simulink model "myGuyton_corrected_new"  (Simulink 6.6)
settings: Solver=ode15s  StartTime=0  StopTime=60*24*14  FixedStep=0.025  MaxStep=1  MinStep=0.00000001  RelTol=1e-1
values from neighbouring files (symbols this model uses):
  A1K = 0.5    [G92_var_decl_exp.m]
  A2K = 60    [G92_var_decl_exp.m]
  A3K = 40000    [G92_var_decl_exp.m]
  A4K = 0.1    [G92_var_decl_exp.m]
  A4K2 = 40000    [G92_var_decl_exp.m]
  AARK = 1    [G92_var_decl_exp.m]
  AARLL = 4    [G92_var_decl_exp.m]
  ADHC_IC = 1.01449    [G92_var_decl_exp.m]
  ADHINF = 0    [G92_var_decl_exp.m]
  ADHKLL = 0.2    [G92_var_decl_exp.m]
  ADHKUL = 5    [G92_var_decl_exp.m]
  ADHPAM = 0.3    [G92_var_decl_exp.m]
  ADHPUL = 85    [G92_var_decl_exp.m]
  ADHTC = 15    [G92_var_decl_exp.m]
  ADHVLL = 0.93617    [G92_var_decl_exp.m]
  ADHVUL = 2.5    [G92_var_decl_exp.m]
  AH10 = 0.333    [G92_var_decl_exp.m]
  AH11 = 1000    [G92_var_decl_exp.m]
  AH9 = 1    [G92_var_decl_exp.m]
  AHMNAR = 0.3    [G92_var_decl_exp.m]
  AHTHM = 2    [G92_var_decl_exp.m]
  AHY_IC = -0.461862    [G92_var_decl_exp.m]
  ALCLK = 0.3    [G92_var_decl_exp.m]
  ALDINF = 0    [G92_var_decl_exp.m]
  ALDKNS = 0    [G92_var_decl_exp.m]
  ALDMM = 2.5    [G92_var_decl_exp.m]
  AM1LL = 0    [G92_var_decl_exp.m]
  AM1UL = 5    [G92_var_decl_exp.m]
  AMC_IC = 1.05537    [G92_var_decl_exp.m]
  AMCSNS = 0.65    [G92_var_decl_exp.m]
  AMKM = 0.5    [G92_var_decl_exp.m]
  AMKMUL = 12    [G92_var_decl_exp.m]
  AMM1_IC = 1.00227    [G92_var_decl_exp.m]
  AMM2_IC = 1.09458    [G92_var_decl_exp.m]
  AMM4 = 0.005    [G92_var_decl_exp.m]
  AMNALL = 0.04    [G92_var_decl_exp.m]
  AMNAM = 0.8    [G92_var_decl_exp.m]
  AMNAUL = 15    [G92_var_decl_exp.m]
  AMT = 60    [G92_var_decl_exp.m]
  ANC_IC = 0.867681    [G92_var_decl_exp.m]
  ANCSNS = 0.4    [G92_var_decl_exp.m]
  ANGINF = 0    [G92_var_decl_exp.m]
  ANGKNS = 0    [G92_var_decl_exp.m]
  ANMALD = 2.5    [G92_var_decl_exp.m]
  ANMAM = 1.4    [G92_var_decl_exp.m]
  ANMARL = 0.86    [G92_var_decl_exp.m]
  ANMEM = 1.6    [G92_var_decl_exp.m]
  ANMKEL = 0.3    [G92_var_decl_exp.m]
  ANMKEM = 2    [G92_var_decl_exp.m]
  ANMLL = 0.7    [G92_var_decl_exp.m]
  ANMNAM = 1    [G92_var_decl_exp.m]
  ANMSLT = 2    [G92_var_decl_exp.m]
  ANMTM = 1.5    [G92_var_decl_exp.m]
  ANMUL = 1.8    [G92_var_decl_exp.m]
  ANPC_IC = 0.9333    [G92_var_decl_exp.m]
  ANPINF = 0    [G92_var_decl_exp.m]
  ANPKNS = 0    [G92_var_decl_exp.m]
  ANPTC = 4    [G92_var_decl_exp.m]
  ANPXAF = 1.5    [G92_var_decl_exp.m]
  ANPXUL = 10    [G92_var_decl_exp.m]
  ANT = 12    [G92_var_decl_exp.m]
  ANULL = 0.8    [G92_var_decl_exp.m]
  ANUM = 6    [G92_var_decl_exp.m]
  ANUVM = 0    [G92_var_decl_exp.m]
  ANV = 5000    [G92_var_decl_exp.m]
  ANX1_IC = 0    [G92_var_decl_exp.m]
  ANXM = 0    [G92_var_decl_exp.m]
  ANY = -0.2    [G92_var_decl_exp.m]
  AR1_IC = 1.00197    [G92_var_decl_exp.m]
  AR2_IC = 1.00306    [G92_var_decl_exp.m]
  AR3_IC = 1.05777    [G92_var_decl_exp.m]
  ARF = 0.5    [G92_var_decl_exp.m]
  ATRFBM = 0    [G92_var_decl_exp.m]
  ATRVM = 0    [G92_var_decl_exp.m]
  AU1_IC = 0.99999    [G92_var_decl_exp.m]
  AU4_IC = -0.00833091    [G92_var_decl_exp.m]
  AU6_IC = 1.00041    [G92_var_decl_exp.m]
  AUC1 = 0.3    [G92_var_decl_exp.m]
  AUDMP = 0.3    [G92_var_decl_exp.m]
  AUK = 0.004    [G92_var_decl_exp.m]
  AUL = 1.5    [G92_var_decl_exp.m]
  AULPM = 0    [G92_var_decl_exp.m]
  AUM1 = 3    [G92_var_decl_exp.m]
  AUM2 = 1    [G92_var_decl_exp.m]
  AUMAX = 5    [G92_var_decl_exp.m]
  AUMIN = 0.4    [G92_var_decl_exp.m]
  AUMK1 = 0.3    [G92_var_decl_exp.m]
  AUN1 = 0.5    [G92_var_decl_exp.m]
  AUS = 1    [G92_var_decl_exp.m]
  AUSLP = 1.5    [G92_var_decl_exp.m]
  AUTOGN = 7    [G92_var_decl_exp.m]
  AUTOK = 0.1    [G92_var_decl_exp.m]
  AUTOSN = 0.9    [G92_var_decl_exp.m]
  AUV = 0.55    [G92_var_decl_exp.m]
  AUX = 1    [G92_var_decl_exp.m]
  AUY = 0    [G92_var_decl_exp.m]
  BAROTC = 0.16    [G92_var_decl_exp.m]
  CFC = 0.01167    [G92_var_decl_exp.m]
  CKEEX = 4    [G92_var_decl_exp.m]
  CMPTSS = 2    [G92_var_decl_exp.m]
  CN2 = 0.0212    [G92_var_decl_exp.m]
  CN3_IC = 0.359907    [G92_var_decl_exp.m]
  CN7 = 0.2    [G92_var_decl_exp.m]
  CNR = 139    [G92_var_decl_exp.m]
  CPF = 0.0003    [G92_var_decl_exp.m]
  CPK = 0.000253    [G92_var_decl_exp.m]
  CPR = 40    [G92_var_decl_exp.m]
  CRRFLX = 0    [G92_var_decl_exp.m]
  CV = 0.1    [G92_var_decl_exp.m]
  DFP_IC = 1.16492e-06    [G92_var_decl_exp.m]
  DHDTR = 0.05    [G92_var_decl_exp.m]
  DIURET = 1    [G92_var_decl_exp.m]
  DR = 0    [G92_var_decl_exp.m]
  DTKA_IC = 0.0368507    [G92_var_decl_exp.m]
  DTNAR = 0.675    [G92_var_decl_exp.m]
  DTNARL = 1e-06    [G92_var_decl_exp.m]
  EARK = 1    [G92_var_decl_exp.m]
  EARLL = 24    [G92_var_decl_exp.m]
  EFAFR = 0    [G92_var_decl_exp.m]
  EXC = 1    [G92_var_decl_exp.m]
  ... (+137 more)
libraries: simulink x5
(part 2 of 3)

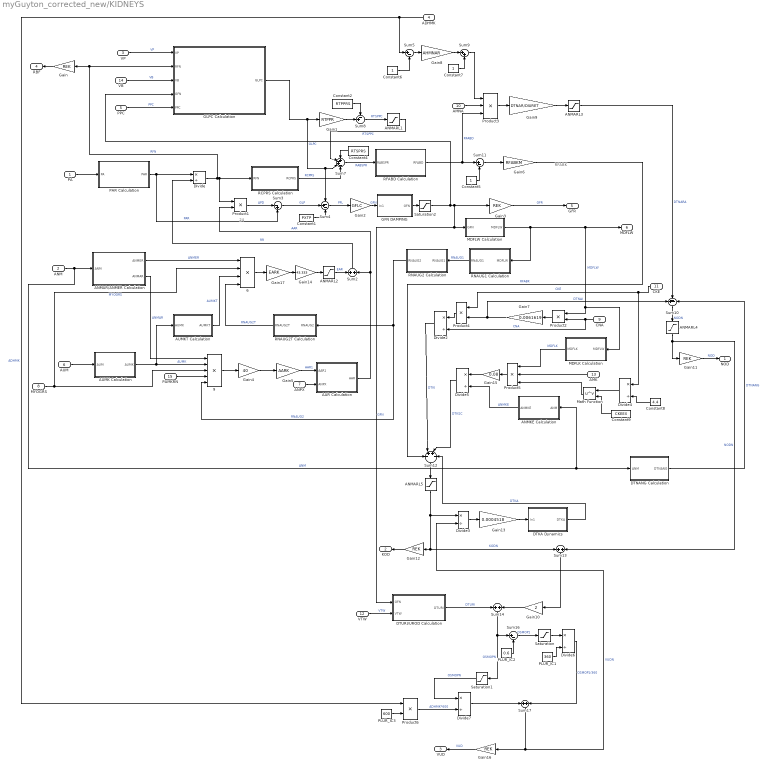
== system myGuyton_corrected_new/KIDNEYS ==
  note: RFABK
  note: 24
  PA : Inport
  ANM : Inport  Port=2
  VP : Inport  Port=3
  ADHMK : Inport  Orientation=left  Port=4
  PPC : Inport  Port=5
  AUM : Inport  Port=6
  ANPX : Inport  Port=7
  MYOGRS : Inport  Port=8
  CNA : Inport  Orientation=left  Port=9
  AMNA : Inport  Port=10
  CKE : Inport  Orientation=left  Port=11
  VTW : Inport  Port=12
  AMK : Inport  Orientation=left  Port=13
  VB : Inport  Port=14
  PAMKRN : Inport  Port=15
  6 : Product  Inputs=4  RndMeth=Zero
  9 : Product  Inputs=5  RndMeth=Zero
  AAR Calculation : Subsystem
  ANMAR/ANMER Calculation : Subsystem
  ANMARL1 : Saturate  UpperLimit=inf  LowerLimit=1
  ANMARL2 : Saturate  UpperLimit=inf  LowerLimit=EARLL
  ANMARL3 : Saturate  UpperLimit=inf  LowerLimit=DTNARL
  ANMARL4 : Saturate  Orientation=down  UpperLimit=inf  LowerLimit=0.00000001
  ANMARL5 : Saturate  Orientation=down  UpperLimit=inf  LowerLimit=0
  ANMKE Calculation : Subsystem  Orientation=left
  AUMK Calculation : Subsystem
  AUMKT Calculation : Subsystem
  Constant1 : Constant  Value=PXTP
  Constant2 : Constant  Value=RTPPRS
  Constant4 : Constant  Orientation=left  Value=RTSPRS
  Constant5 : Constant
  Constant6 : Constant
  Constant7 : Constant
  Constant8 : Constant  Orientation=left  Value=4.4
  Constant9 : Constant  Orientation=left  Value=CKEEX
  DTKA Dynamics : Subsystem
      mask Display: dpoly([0 1],[1 1])
  DTNANG Calculation : Subsystem
  DTURI/UROD Calculation : Subsystem
  Divide{,3,6..7} (4 alike) : Product  Inputs=*/  OutScaling=2^-10
  Divide2 : Product  Orientation=left  Inputs=*/  OutScaling=2^-10
  Divide4 : Product  Orientation=left  Inputs=*/  OutScaling=2^-10
  Divide5 : Product  Orientation=left  Inputs=*/  OutScaling=2^-10
  GFN DAMPING : Subsystem
      mask Display: dpoly([0 1],[GFNDMP 1])
  GLPC Calculation : Subsystem
  Gain : Gain  Orientation=left  Gain=REK
  Gain1 : Gain  Gain=RTPPR
  Gain10 : Gain  Orientation=left  Gain=2
  Gain11 : Gain  Gain=REK
  Gain12 : Gain  Orientation=left  Gain=REK
  Gain13 : Gain  Gain=0.0004518
  Gain14 : Gain  Gain=43.333
  Gain15 : Gain  Orientation=left  Gain=0.08
  Gain16 : Gain  Orientation=left  Gain=REK
  Gain17 : Gain  Gain=EARK
  Gain2 : Gain  Gain=GFLC
  Gain3 : Gain  Gain=REK
  Gain4 : Gain  Gain=40
  Gain5 : Gain  Gain=AARK
  Gain6 : Gain  Gain=RFABKM
  Gain7 : Gain  Orientation=left  Gain=0.0061619
  Gain8 : Gain  Gain=AHMNAR
  Gain9 : Gain  Gain=DTNAR/DIURET
  MDFLK Calculation : Subsystem  Orientation=left
  MDFLW Calculation : Subsystem
  Math Function : Math  Orientation=left  Operator=pow  SaturateOnIntegerOverflow=on
  PAR Calculation : Subsystem
  PLUR_IC1 : Constant  Value=360
  PLUR_IC2 : Constant  Value=0.6
  PLUR_IC3 : Constant  Value=600
  Product1 : Product  RndMeth=Zero
  Product2 : Product  Orientation=left  RndMeth=Zero
  Product3 : Product  Inputs=3  RndMeth=Zero
  Product4 : Product  Orientation=left  RndMeth=Zero
  Product5 : Product  Orientation=left  Inputs=3  RndMeth=Zero
  Product6 : Product  RndMeth=Zero
  RCPRS Calculation : Subsystem
  RFABD Calculation : Subsystem
  RNAUG1 Calculation : Subsystem  Orientation=left
  RNAUG2 Calculation : Subsystem  Orientation=left
  RNAUG2T Calculation : Subsystem  Orientation=left
  Saturation : Saturate  UpperLimit=inf  LowerLimit=0
  Saturation1 : Saturate  Orientation=left  UpperLimit=0.6  LowerLimit=-inf
  Saturation2 : Saturate  UpperLimit=inf  LowerLimit=GFNLL
  Sum10 : Sum  Orientation=down  Inputs=+--
  Sum11 : Sum  Inputs=|+-
  Sum12 : Sum  Orientation=down  Inputs=-++-
  Sum13 : Sum  Orientation=down
  Sum14 : Sum  Orientation=down
  Sum16 : Sum  Inputs=|+-
  Sum17 : Sum  Orientation=down
  Sum2 : Sum  Orientation=up
  Sum3 : Sum  Inputs=|-+
  Sum4 : Sum  Inputs=-+-
  Sum5 : Sum  Inputs=|+-
  Sum7 : Sum  Inputs=+-+-
  Sum8 : Sum  Inputs=-+|
  Sum9 : Sum  Inputs=|++
  NOD : Outport
  KOD : Outport  Orientation=left  Port=2
  VUD : Outport  Orientation=left  Port=3
  RBF : Outport  Orientation=left  Port=4
  GFR : Outport  Port=5
  MDFLW : Outport  Port=6
  wires:
  PAR Calculation/1(PAR) -> Divide/1, Sum3/2  "PAR"
  PA/1 -> PAR Calculation/1(PA)
  Divide/1 -> RCPRS Calculation/1(RFN), Product1/1, Gain/1, GLPC Calculation/2(RFN)  "RFN"
  Gain/1 -> RBF/1
  ANMAR/ANMER Calculation/1(ANMER) -> 6/1  "ANMER"
  RCPRS Calculation/1(RCPRS) -> Sum7/4  "RCPRS"
  AUM/1 -> AUMK Calculation/1(AUM)
  AUMK Calculation/1(AUMK) -> 9/2, AUMKT Calculation/1(AUMK)  "AUMK"
  GLPC Calculation/1(GLPC) -> Gain1/1, Sum7/3, Sum4/1  "GLPC"
  Constant2/1 -> Sum8/1
  Gain1/1 -> Sum8/2
  Sum8/1 -> ANMARL1/1  "RTSPPC"
  ANMARL1/1 -> Sum7/2  "RTSPPC"
  Constant4/1 -> Sum7/1
  Sum7/1 -> RFABD Calculation/1(RABSPR)  "RABSPR"
  RFABD Calculation/1(RFABD) -> Sum11/1, Product3/3  "RFABD"
  Sum11/1 -> Gain6/1
  Constant5/1 -> Sum11/2
  Gain6/1 -> Sum12/1  "RFABK"
  ANMAR/ANMER Calculation/2(ANMAR) -> 9/1  "ANMAR"
  9/1 -> Gain4/1
  Gain4/1 -> Gain5/1
  Gain5/1 -> AAR Calculation/1(AAR1)  "AAR1"
  MYOGRS/1 -> 9/3, 6/2  "MYOGRS"
  AAR Calculation/1(AAR) -> Product1/2, Sum2/2  "AAR"
  ANPX/1 -> AAR Calculation/2(ANPX)
  ANM/1 -> ANMAR/ANMER Calculation/1(ANM), ANMKE Calculation/1(ANM), DTNANG Calculation/1(ANM)  "ANM"
  AUMKT Calculation/1(AUMKT) -> 6/3  "AUMKT"
  RNAUG2T Calculation/1(RNAUG2T) -> 6/4  "RNAUG2T"
  ANMARL2/1 -> Sum2/1  "EAR"
  Sum2/1 -> Divide/2  "RR"
  Product1/1 -> Sum3/1  "APD"
  Sum3/1 -> Sum4/2  "GLP"
  Constant1/1 -> Sum4/3
  Sum4/1 -> Gain2/1  "PFL"
  Gain2/1 -> GFN DAMPING/1(In1)  "GFN"
  Gain3/1 -> GFR/1  "GFR"
  MDFLW Calculation/1(MDFLW) -> RNAUG1 Calculation/1(MDFLW), MDFLW/1, Product2/1, MDFLK Calculation/1(MDFLW)  "MDFLW"
  RNAUG1 Calculation/1(RNAUG1) -> RNAUG2 Calculation/1(RNAUG1)  "RNAUG1"
  RNAUG2 Calculation/1(RNAUG2) -> RNAUG2T Calculation/1(RNAUG2), 9/5  "RNAUG2"
  CNA/1 -> Product2/2, Divide2/2  "CNA"
  Product2/1 -> Gain7/1
  Gain7/1 -> Product4/2, Sum10/1  "DTNAI"
  AMNA/1 -> Product3/2
  ADHMK/1 -> Sum5/1, Product6/1  "ADHMK"
  Constant6/1 -> Sum5/2
  Sum5/1 -> Gain8/1
  Gain8/1 -> Sum9/1
  Constant7/1 -> Sum9/2
  Sum9/1 -> Product3/1
  Product3/1 -> Gain9/1
  Gain9/1 -> ANMARL3/1
  CKE/1 -> Product4/1, Divide4/1  "CKE"
  Product4/1 -> Divide2/1
  Divide2/1 -> Sum12/2  "DTKI"
  ANMARL3/1 -> Sum10/2  "DTNARA"
  Sum10/1 -> ANMARL4/1  "NODN"
  Gain11/1 -> NOD/1  "NOD"
  Divide5/1 -> Sum12/3  "DTKSC"
  Sum12/1 -> ANMARL5/1
  ANMARL5/1 -> Sum13/1, Gain12/1, Divide3/1  "KODN"
  DTNANG Calculation/1(DTNANG) -> Sum10/3  "DTNANG"
  Sum13/1 -> Gain10/1
  Gain12/1 -> KOD/1
  Gain10/1 -> Sum14/2
  Divide3/1 -> Gain13/1
  Gain13/1 -> DTKA Dynamics/1(In1)
  DTKA Dynamics/1(DTKA) -> Sum12/4  "DTKA"
  Sum14/1 -> Sum16/1, Saturation1/1  "OSMOPN"
  PLUR_IC2/1 -> Sum16/2
  Sum16/1 -> Saturation/1  "OSMOP1"
  Saturation1/1 -> Divide7/1  "OSMOPN"
  Saturation/1 -> Divide6/1
  PLUR_IC1/1 -> Divide6/2
  Divide6/1 -> Sum17/2  "OSMOP1/360"
  Sum17/1 -> Divide3/2, Gain16/1  "VUDN"
  PLUR_IC3/1 -> Product6/2
  Product6/1 -> Divide7/2  "ADHMK*600"
  Divide7/1 -> Sum17/1
  Gain16/1 -> VUD/1  "VUD"
  DTURI/UROD Calculation/1(DTURI) -> Sum14/1  "DTURI"
  VTW/1 -> DTURI/UROD Calculation/2(VTW)  "VTW"
  Constant8/1 -> Divide4/2
  Divide4/1 -> Math Function/1
  Constant9/1 -> Math Function/2
  Math Function/1 -> Product5/3
  AMK/1 -> Product5/2
  MDFLK Calculation/1(MDFLK) -> Product5/1  "MDFLK"
  Product5/1 -> Gain15/1
  Gain15/1 -> Divide5/1
  ANMKE Calculation/1(ANMKE) -> Divide5/2  "ANMKE"
  VP/1 -> GLPC Calculation/1(VP)  "VP"
  VB/1 -> GLPC Calculation/3(VB)  "VB"
  PPC/1 -> GLPC Calculation/5(PPC)  "PPC"
  PAMKRN/1 -> 9/4
  Gain14/1 -> ANMARL2/1
  6/1 -> Gain17/1
  Gain17/1 -> Gain14/1
  ANMARL4/1 -> Sum13/2, Gain11/1  "NODN"
  Saturation2/1 -> Gain3/1, MDFLW Calculation/1(GFN), DTURI/UROD Calculation/1(GFN), GLPC Calculation/4(GFN)  "GFN"
  GFN DAMPING/1(GFN) -> Saturation2/1

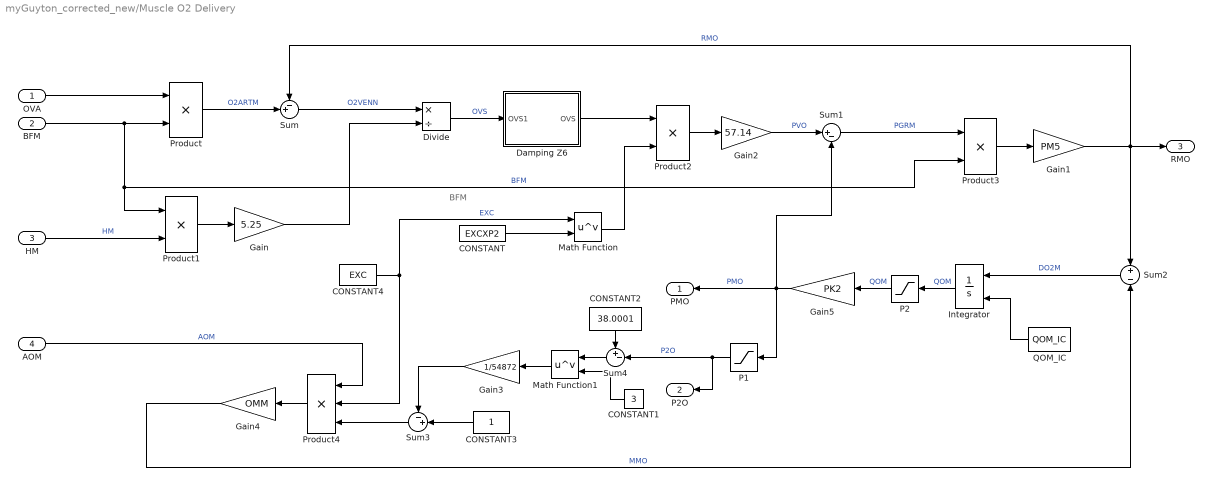
== system myGuyton_corrected_new/Muscle O2 Delivery ==
  note: BFM
  OVA : Inport
  BFM : Inport  Port=2
  HM : Inport  Port=3
  AOM : Inport  Port=4
  CONSTANT : Constant  Value=EXCXP2
  CONSTANT1 : Constant  Orientation=left  Value=3
  CONSTANT2 : Constant  Orientation=down  Value=38.0001
  CONSTANT3 : Constant  Orientation=left
  CONSTANT4 : Constant  Value=EXC
  Damping Z6 : Subsystem
      mask Display: dpoly([0 1], [Z6 1])
  Divide : Product  Inputs=*/  OutScaling=2^-10
  Gain : Gain  Gain=5.25
  Gain1 : Gain  Gain=PM5
  Gain2 : Gain  Gain=57.14
  Gain3 : Gain  Orientation=left  Gain=1/54872
  Gain4 : Gain  Orientation=left  Gain=OMM
  Gain5 : Gain  Orientation=left  Gain=PK2
  Integrator : Integrator  Orientation=left  InitialConditionSource=external
  Math Function : Math  Operator=pow  SaturateOnIntegerOverflow=on
  Math Function1 : Math  Orientation=left  Operator=pow  SaturateOnIntegerOverflow=on
  P1 : Saturate  Orientation=left  UpperLimit=38  LowerLimit=-inf
  P2 : Saturate  Orientation=left  UpperLimit=inf  LowerLimit=0.0001
  Product{,1..3} (4 alike) : Product  RndMeth=Zero
  Product4 : Product  Orientation=left  Inputs=3  RndMeth=Zero
  QOM_IC : Constant  Orientation=left  Value=QOM_IC
  Sum : Sum  Inputs=-+|
  Sum1 : Sum  Inputs=|+-
  Sum2 : Sum  Orientation=left  Inputs=+-
  Sum3 : Sum  Orientation=left  Inputs=-+|
  Sum4 : Sum  Orientation=left  Inputs=+-|
  PMO : Outport  Orientation=left
  P2O : Outport  Orientation=left  Port=2
  RMO : Outport  Port=3
  wires:
  Divide/1 -> Damping Z6/1(OVS1)  "OVS"
  Product/1 -> Sum/2  "O2ARTM"
  Sum/1 -> Divide/1  "O2VENN"
  Gain/1 -> Divide/2
  Product1/1 -> Gain/1
  HM/1 -> Product1/2  "HM"
  BFM/1 -> Product/2, Product1/1, Product3/2  "BFM"
  OVA/1 -> Product/1
  CONSTANT/1 -> Math Function/2
  Math Function/1 -> Product2/2
  Product2/1 -> Gain2/1
  Product3/1 -> Gain1/1
  Gain1/1 -> Sum/1, Sum2/1, RMO/1  "RMO"
  Sum2/1 -> Integrator/1  "DO2M"
  QOM_IC/1 -> Integrator/2
  Integrator/1 -> P2/1  "QOM"
  P2/1 -> Gain5/1  "QOM"
  Gain5/1 -> Sum1/2, PMO/1, P1/1  "PMO"
  Gain2/1 -> Sum1/1  "PVO"
  Sum1/1 -> Product3/1  "PGRM"
  P1/1 -> Sum4/2, P2O/1  "P2O"
  CONSTANT2/1 -> Sum4/1
  Sum4/1 -> Math Function1/1
  CONSTANT1/1 -> Math Function1/2
  Math Function1/1 -> Gain3/1
  CONSTANT3/1 -> Sum3/2
  Gain3/1 -> Sum3/1
  Sum3/1 -> Product4/3
  AOM/1 -> Product4/1  "AOM"
  Product4/1 -> Gain4/1
  Gain4/1 -> Sum2/2  "MMO"
  CONSTANT4/1 -> Math Function/1, Product4/2  "EXC"
  Damping Z6/1(OVS) -> Product2/1

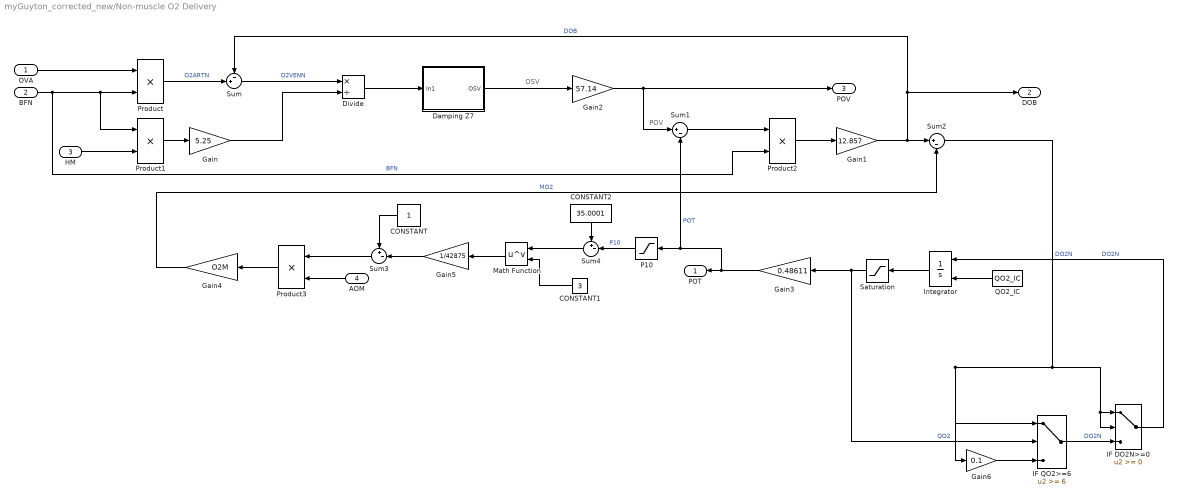
== system myGuyton_corrected_new/Non-muscle O2 Delivery ==
  note: POV
  note: OSV
  OVA : Inport
  BFN : Inport  Port=2
  HM : Inport  Port=3
  AOM : Inport  Orientation=left  Port=4
  CONSTANT : Constant  Orientation=left
  CONSTANT1 : Constant  Orientation=left  Value=3
  CONSTANT2 : Constant  Orientation=down  Value=35.0001
  Damping Z7 : Subsystem
      mask Display: dpoly([0 1], [Z7 1])
  Divide : Product  Inputs=*/  OutScaling=2^-10
  Gain : Gain  Gain=5.25
  Gain1 : Gain  Gain=12.857
  Gain2 : Gain  Gain=57.14
  Gain3 : Gain  Orientation=left  Gain=0.48611
  Gain4 : Gain  Orientation=left  Gain=O2M
  Gain5 : Gain  Orientation=left  Gain=1/42875
  Gain6 : Gain  Gain=0.1
  IF DO2N>=0 : Switch
  IF QO2>=6 : Switch  Threshold=6
  Integrator : Integrator  Orientation=left  InitialConditionSource=external
  Math Function : Math  Orientation=left  Operator=pow  SaturateOnIntegerOverflow=on
  P10 : Saturate  Orientation=left  UpperLimit=35  LowerLimit=-inf
  Product : Product  RndMeth=Zero
  Product1 : Product  RndMeth=Zero
  Product2 : Product  RndMeth=Zero
  Product3 : Product  Orientation=left  RndMeth=Zero
  QO2_IC : Constant  Orientation=left  Value=QO2_IC
  Saturation : Saturate  Orientation=left  UpperLimit=inf  LowerLimit=0
  Sum : Sum  Inputs=-+|
  Sum1 : Sum  Inputs=|+-
  Sum2 : Sum  Inputs=|+-
  Sum3 : Sum  Orientation=left  Inputs=+-|
  Sum4 : Sum  Orientation=left  Inputs=+-|
  POT : Outport  Orientation=left
  DOB : Outport  Port=2
  POV : Outport  Port=3
  wires:
  OVA/1 -> Product/1
  BFN/1 -> Product/2, Product1/1, Product2/2  "BFN"
  HM/1 -> Product1/2
  Product1/1 -> Gain/1
  Gain/1 -> Divide/2
  Sum/1 -> Divide/1  "O2VENN"
  Product/1 -> Sum/2  "O2ARTN"
  Divide/1 -> Damping Z7/1(In1)
  Gain2/1 -> POV/1, Sum1/1
  Sum1/1 -> Product2/1
  Product2/1 -> Gain1/1
  Gain1/1 -> Sum2/1, Sum/1, DOB/1  "DOB"
  Sum2/1 -> IF QO2>=6/1, Gain6/1, IF DO2N>=0/1, IF DO2N>=0/2  "DO2N"
  QO2_IC/1 -> Integrator/2
  Integrator/1 -> Saturation/1
  Saturation/1 -> Gain3/1, IF QO2>=6/2  "QO2"
  Gain3/1 -> POT/1, Sum1/2, P10/1  "POT"
  Product3/1 -> Gain4/1
  Gain4/1 -> Sum2/2  "MO2"
  AOM/1 -> Product3/2
  Gain5/1 -> Sum3/2
  Sum3/1 -> Product3/1
  Math Function/1 -> Gain5/1
  CONSTANT1/1 -> Math Function/2
  P10/1 -> Sum4/2  "P10"
  CONSTANT2/1 -> Sum4/1
  Sum4/1 -> Math Function/1
  CONSTANT/1 -> Sum3/1
  Gain6/1 -> IF QO2>=6/3
  IF QO2>=6/1 -> IF DO2N>=0/3  "DO2N"
  IF DO2N>=0/1 -> Integrator/1  "DO2N"
  Damping Z7/1(OSV) -> Gain2/1

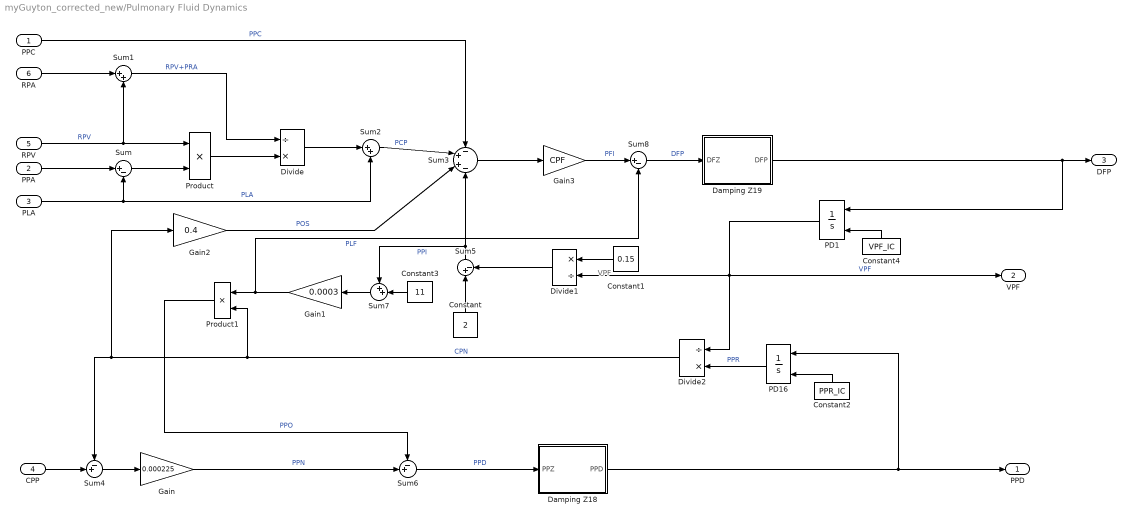
== system myGuyton_corrected_new/Pulmonary Fluid Dynamics ==
  note: VPF
  PPC : Inport
  PPA : Inport  Port=2
  PLA : Inport  Port=3
  CPP : Inport  Port=4
  RPV : Inport  Port=5
  RPA : Inport  Port=6
  Constant : Constant  Orientation=up  Value=2
  Constant1 : Constant  Orientation=left  Value=0.15
  Constant2 : Constant  Orientation=up  Value=PPR_IC
  Constant3 : Constant  Orientation=left  Value=11
  Constant4 : Constant  Orientation=up  Value=VPF_IC
  Damping Z18 : Subsystem
      mask Display: dpoly([0 1],[Z18 1])
  Damping Z19 : Subsystem
      mask Display: dpoly([0 1],[Z19 1])
  Divide : Product  Inputs=/*  OutScaling=2^-10
  Divide1 : Product  Orientation=left  Inputs=*/  OutScaling=2^-10
  Divide2 : Product  Orientation=left  Inputs=/*  OutScaling=2^-10
  Gain : Gain  Gain=0.000225
  Gain1 : Gain  Orientation=left  Gain=0.0003
  Gain2 : Gain  Gain=0.4
  Gain3 : Gain  Gain=CPF
  PD1 : Integrator  Orientation=left  InitialConditionSource=external
  PD16 : Integrator  Orientation=left  InitialConditionSource=external
  Product : Product  RndMeth=Zero
  Product1 : Product  Orientation=left  RndMeth=Zero
  Sum : Sum  Inputs=|+-
  Sum1 : Sum  Inputs=|++
  Sum2 : Sum  Inputs=|++
  Sum3 : Sum  Inputs=-++-
  Sum4 : Sum  Inputs=-+|
  Sum5 : Sum  Orientation=up  Inputs=|+-
  Sum6 : Sum  Inputs=-+|
  Sum7 : Sum  Orientation=left  Inputs=++|
  Sum8 : Sum  Inputs=|+-
  PPD : Outport
  VPF : Outport  Port=2
  DFP : Outport  Port=3
  wires:
  PLA/1 -> Sum/2, Sum2/2  "PLA"
  PPA/1 -> Sum/1
  RPV/1 -> Product/1, Sum1/2  "RPV"
  Sum/1 -> Product/2
  RPA/1 -> Sum1/1
  Product/1 -> Divide/2
  Sum1/1 -> Divide/1  "RPV+PRA"
  Divide/1 -> Sum2/1
  PPC/1 -> Sum3/1  "PPC"
  Sum2/1 -> Sum3/2  "PCP"
  Sum5/1 -> Sum3/4, Sum7/1  "PPI"
  Sum3/1 -> Gain3/1
  Constant/1 -> Sum5/1
  Constant1/1 -> Divide1/1
  Divide1/1 -> Sum5/2
  Sum4/1 -> Gain/1
  Sum6/1 -> Damping Z18/1(PPZ)  "PPD"
  Constant2/1 -> PD16/2
  PD16/1 -> Divide2/2  "PPR"
  Divide2/1 -> Product1/2, Sum4/1, Gain2/1  "CPN"
  CPP/1 -> Sum4/2
  Constant3/1 -> Sum7/2
  Sum7/1 -> Gain1/1
  Gain1/1 -> Product1/1, Sum8/2  "PLF"
  Product1/1 -> Sum6/1  "PPO"
  Gain2/1 -> Sum3/3  "POS"
  Gain3/1 -> Sum8/1  "PFI"
  Sum8/1 -> Damping Z19/1(DFZ)  "DFP"
  PD1/1 -> Divide2/1, VPF/1, Divide1/2  "VPF"
  Gain/1 -> Sum6/2  "PPN"
  Constant4/1 -> PD1/2
  Damping Z18/1(PPD) -> PPD/1, PD16/1
  Damping Z19/1(DFP) -> PD1/1, DFP/1

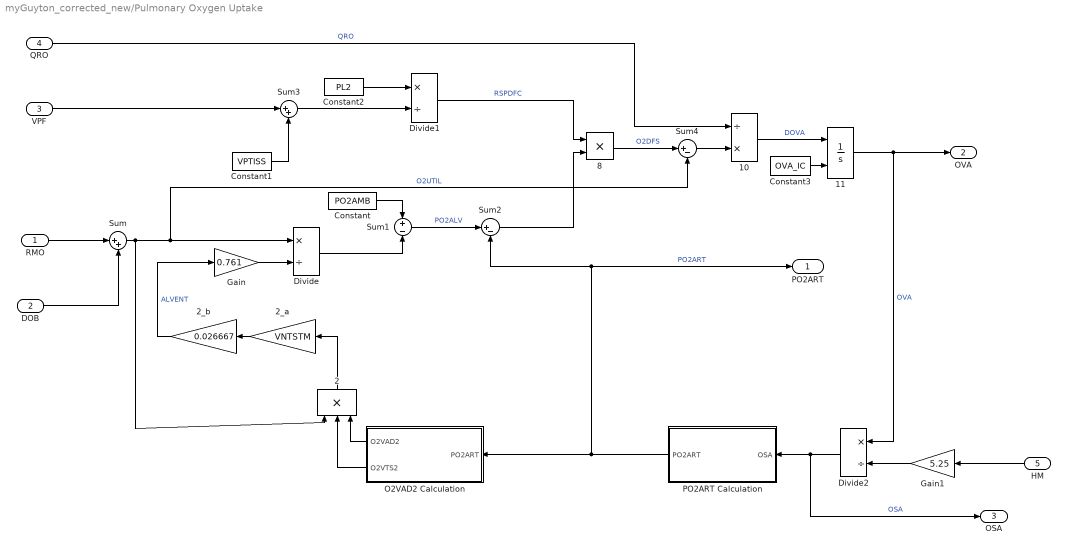
== system myGuyton_corrected_new/Pulmonary Oxygen Uptake ==
  RMO : Inport
  DOB : Inport  Port=2
  VPF : Inport  Port=3
  QRO : Inport  Port=4
  HM : Inport  Orientation=left  Port=5
  10 : Product  Inputs=/*  OutScaling=2^-10  RndMeth=Nearest
  11 : Integrator  InitialConditionSource=external
  2 : Product  Orientation=up  Inputs=3  RndMeth=Zero
  2_a : Gain  Orientation=left  Gain=VNTSTM
  2_b : Gain  Orientation=left  Gain=0.026667
  8 : Product  RndMeth=Zero
  Constant : Constant  Value=PO2AMB
  Constant1 : Constant  Value=VPTISS
  Constant2 : Constant  Value=PL2
  Constant3 : Constant  Value=OVA_IC
  Divide : Product  Inputs=*/  OutScaling=2^-10
  Divide1 : Product  Inputs=*/  OutScaling=2^-10
  Divide2 : Product  Orientation=left  Inputs=*/  OutScaling=2^-10
  Gain : Gain  Gain=0.761
  Gain1 : Gain  Orientation=left  Gain=5.25
  O2VAD2 Calculation : Subsystem  Orientation=left
  PO2ART Calculation : Subsystem  Orientation=left
  Sum : Sum  Inputs=|++
  Sum1 : Sum  Inputs=+-
  Sum2 : Sum  Inputs=|+-
  Sum3 : Sum  Inputs=|++
  Sum4 : Sum  Inputs=|+-
  PO2ART : Outport
  OVA : Outport  Port=2
  OSA : Outport  Port=3
  wires:
  RMO/1 -> Sum/1
  DOB/1 -> Sum/2
  Sum/1 -> Divide/1, Sum4/2, 2/1  "O2UTIL"
  Gain/1 -> Divide/2
  2_b/1 -> Gain/1  "ALVENT"
  Divide/1 -> Sum1/2
  Constant/1 -> Sum1/1
  Sum1/1 -> Sum2/1  "PO2ALV"
  Sum2/1 -> 8/2
  VPF/1 -> Sum3/1
  Constant1/1 -> Sum3/2
  Constant2/1 -> Divide1/1
  Sum3/1 -> Divide1/2
  Divide1/1 -> 8/1  "RSPDFC"
  8/1 -> Sum4/1  "O2DFS"
  Sum4/1 -> 10/2
  QRO/1 -> 10/1  "QRO"
  10/1 -> 11/1  "DOVA"
  11/1 -> OVA/1, Divide2/1  "OVA"
  HM/1 -> Gain1/1
  Gain1/1 -> Divide2/2
  Divide2/1 -> PO2ART Calculation/1(OSA), OSA/1  "OSA"
  PO2ART Calculation/1(PO2ART) -> Sum2/2, PO2ART/1, O2VAD2 Calculation/1(PO2ART)  "PO2ART"
  2/1 -> 2_a/1
  O2VAD2 Calculation/1(O2VAD2) -> 2/3
  2_a/1 -> 2_b/1
  O2VAD2 Calculation/2(O2VTS2) -> 2/2
  Constant3/1 -> 11/2

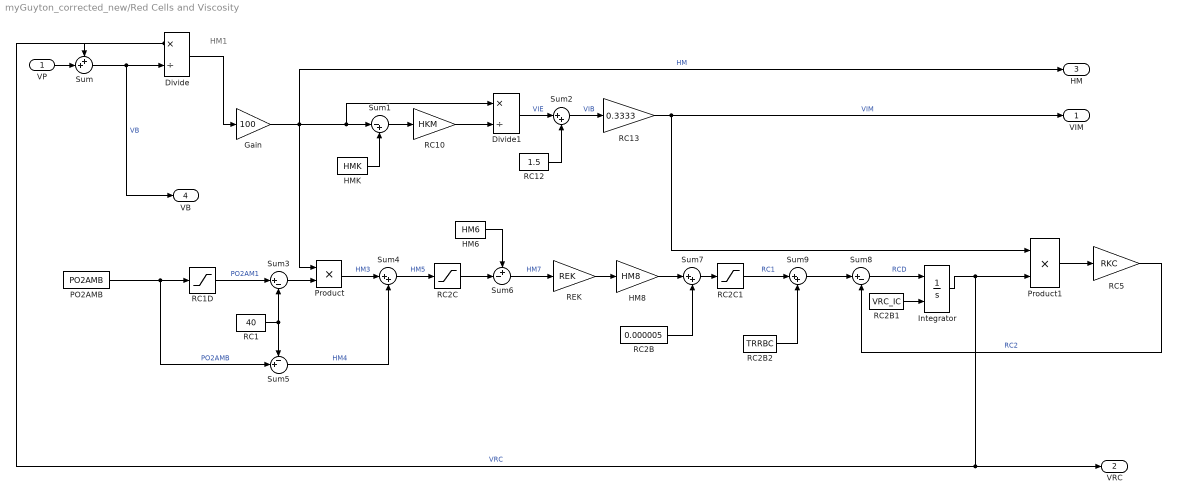
== system myGuyton_corrected_new/Red Cells and Viscosity ==
  note: HM1
  VP : Inport
  Divide : Product  Inputs=*/  OutScaling=2^-10
  Divide1 : Product  Inputs=*/  OutScaling=2^-10
  Gain : Gain  Gain=100
  HM6 : Constant  Value=HM6
  HM8 : Gain  Gain=HM8
  HMK : Constant  Value=HMK
  Integrator : Integrator  InitialConditionSource=external
  PO2AMB : Constant  Value=PO2AMB
  Product : Product  RndMeth=Zero
  Product1 : Product  RndMeth=Zero
  RC1 : Constant  Value=40
  RC10 : Gain  Gain=HKM
  RC12 : Constant  Value=1.5
  RC13 : Gain  Gain=0.3333
  RC1D : Saturate  UpperLimit=80  LowerLimit=-inf  LinearizeAsGain=off
  RC2B : Constant  Value=0.000005
  RC2B1 : Constant  Value=VRC_IC
  RC2B2 : Constant  Value=TRRBC
  RC2C : Saturate  UpperLimit=inf  LowerLimit=0  LinearizeAsGain=off
  RC2C1 : Saturate  UpperLimit=inf  LowerLimit=0  LinearizeAsGain=off
  RC5 : Gain  Gain=RKC
  REK : Gain  Gain=REK
  Sum : Sum  Inputs=++|  OutDataTypeMode=single
  Sum1 : Sum  Inputs=|-+
  Sum{2,4,7,9} (4 alike) : Sum  Inputs=|++
  Sum3 : Sum  Inputs=|+-
  Sum5 : Sum  Inputs=-+|
  Sum6 : Sum  Inputs=+-|
  Sum8 : Sum  Inputs=|+-
  VIM : Outport
  VRC : Outport  Port=2
  HM : Outport  Port=3
  VB : Outport  Port=4
  wires:
  PO2AMB/1 -> RC1D/1, Sum5/2  "PO2AMB"
  RC1D/1 -> Sum3/1  "PO2AM1"
  RC1/1 -> Sum3/2, Sum5/1
  Sum3/1 -> Product/2
  Product/1 -> Sum4/1  "HM3"
  Sum5/1 -> Sum4/2  "HM4"
  RC2C/1 -> Sum6/2
  HM6/1 -> Sum6/1
  Sum6/1 -> REK/1  "HM7"
  REK/1 -> HM8/1
  RC2B/1 -> Sum7/2
  HM8/1 -> Sum7/1
  Sum8/1 -> Integrator/1  "RCD"
  Integrator/1 -> Product1/2, VRC/1, Divide/1, Sum/1  "VRC"
  Sum4/1 -> RC2C/1  "HM5"
  Product1/1 -> RC5/1
  RC5/1 -> Sum8/2  "RC2"
  RC2B1/1 -> Integrator/2
  VP/1 -> Sum/2
  RC13/1 -> VIM/1, Product1/1  "VIM"
  Sum2/1 -> RC13/1  "VIB"
  RC12/1 -> Sum2/2
  Divide1/1 -> Sum2/1  "VIE"
  RC10/1 -> Divide1/2
  Sum1/1 -> RC10/1
  HMK/1 -> Sum1/2
  Gain/1 -> Sum1/1, Divide1/1, HM/1, Product/1  "HM"
  Divide/1 -> Gain/1
  Sum/1 -> Divide/2, VB/1  "VB"
  Sum7/1 -> RC2C1/1
  RC2C1/1 -> Sum9/1  "RC1"
  Sum9/1 -> Sum8/1
  RC2B2/1 -> Sum9/2

== system myGuyton_corrected_new/Thirst, Drinking snd Salt Apetite ==
  note: TVZ+DR
  note: AHTH
  POT : Inport
  ANM : Inport  Port=2
  ADHC : Inport  Port=3
  1 : Saturate  UpperLimit=inf  LowerLimit=0
  AHTH Calculation : Subsystem
      mask Display: disp('AHTH CALCULATION')
  ANMTH Calculation : Subsystem
      mask Display: disp('ANMTH CALCULATION')
  Constant : Constant  Value=DR
  STH Calculation : Subsystem
      mask Display: disp('STH CALCULATION')
  Sum2 : Sum  Inputs=|++
  Sum5 : Sum  Inputs=|++
  TVDDynamics : Subsystem
      mask Display: dpoly([0 1], [TVDDL 1])
  STH : Outport
  TVD : Outport  Port=2
  wires:
  ANM/1 -> STH Calculation/2(ANM), ANMTH Calculation/1(ANM)  "ANM"
  ANMTH Calculation/1(ANMTH) -> Sum5/2  "ANMTH"
  AHTH Calculation/1(AHTH) -> Sum5/1
  Sum5/1 -> 1/1
  STH Calculation/1(STH) -> AHTH Calculation/2(STH), STH/1  "STH"
  1/1 -> Sum2/2  "TVZ"
  Constant/1 -> Sum2/1
  Sum2/1 -> TVDDynamics/1(TVZ+DR)
  POT/1 -> STH Calculation/1(POT)
  TVDDynamics/1(TVD) -> TVD/1
  ADHC/1 -> AHTH Calculation/1(ADHC)  "ADHC"

== system myGuyton_corrected_new/Vascular Stress Relaxation ==
  VVE : Inport
  Constant : Constant  Value=0.74
  SR2 : Gain  Gain=SR
  SR2A : Gain  Gain=SR2
  Sum : Sum  Inputs=|+-
  Sum1 : Sum  Inputs=-+|
  VSR Long Term : Subsystem  Description=Traansfer Function
      mask Display: dpoly([0 1],[SRK2 1],'s')
  VSR Short Term : Subsystem
      mask Display: dpoly([0 1], [SRK 1], 's')
  VV6 : Outport
  VV7 : Outport  Port=2
  wires:
  VVE/1 -> Sum/1, Sum1/2
  Sum/1 -> SR2A/1
  SR2A/1 -> VSR Long Term/1(In1)
  Sum1/1 -> SR2/1
  SR2/1 -> VSR Short Term/1(In1)
  Constant/1 -> Sum/2, Sum1/1
  VSR Long Term/1(VV6) -> VV6/1
  VSR Short Term/1(VV7) -> VV7/1

== system myGuyton_corrected_new/Volume Receptors ==
  note: AHZ_a
  PRA : Inport
  Abs : Abs
  Constant : Constant  Value=AH10
  Constant1 : Constant
  Gain : Gain  Gain=-1
  Math Function : Math  Operator=pow  SaturateOnIntegerOverflow=on
  Sum1 : Sum  Inputs=|+-
  Sum2 : Sum  Inputs=|++
  Switch : Switch
  VR2 : Gain  Gain=AH9
  VR7 : Gain  Gain=ATRFBM
  VR9 : Gain  Gain=ATRVM
  Volume Receptor Adaptation : Subsystem
      mask Display: dpoly([0 1], [AH11 1])
  ATRVFB : Outport
  ATRRFB : Outport  Port=2
  wires:
  PRA/1 -> Abs/1, Switch/2
  Abs/1 -> Math Function/1
  Constant/1 -> Math Function/2
  Math Function/1 -> Gain/1, Switch/1  "AHZ"
  Gain/1 -> Switch/3  "-AHZ"
  Switch/1 -> VR2/1
  VR2/1 -> Sum1/1, Volume Receptor Adaptation/1(AHZ_a)
  Volume Receptor Adaptation/1(AHY) -> Sum1/2  "AHY"
  Sum1/1 -> VR7/1, VR9/1  "AH7"
  VR7/1 -> Sum2/1
  Constant1/1 -> Sum2/2
  VR9/1 -> ATRVFB/1
  Sum2/1 -> ATRRFB/1

== system myGuyton_corrected_new/ADH/ADH (TOTAL ADH SECRETION) ==
  PA1 : Inport
  CNA : Inport  Port=2
  Constant : Constant  Value=CNR
  Constant1 : Constant  Value=142
  Constant2 : Constant  Value=ADHPUL
  Constant3 : Constant  Value=ADHINF
  Divide : Product  Inputs=*/  OutScaling=2^-10
  Gain : Gain  Gain=ADHPAM
  Math Function : Math  Operator=square  SaturateOnIntegerOverflow=on
  Saturation : Saturate  UpperLimit=inf  LowerLimit=0  LinearizeAsGain=off
  Saturation1 : Saturate  UpperLimit=inf  LowerLimit=0  LinearizeAsGain=off
  Saturation2 : Saturate  UpperLimit=ADHPUL  LowerLimit=-inf  LinearizeAsGain=off
  Sum : Sum  Inputs=|+-
  Sum1 : Sum  Inputs=|-+
  Sum2 : Sum  Inputs=|+-
  Sum3 : Sum  Inputs=+++
  ADH : Outport
  wires:
  Constant/1 -> Sum/2, Sum1/1
  Constant1/1 -> Sum1/2
  Sum/1 -> Divide/1
  Sum1/1 -> Divide/2
  Divide/1 -> Saturation/1  "ADHNA"
  Constant2/1 -> Sum2/1  "ADHUL"
  Saturation2/1 -> Sum2/2  "ADHPA"
  Sum2/1 -> Math Function/1
  Math Function/1 -> Gain/1
  Gain/1 -> Sum3/1  "ADHPR"
  Saturation/1 -> Sum3/3  "ADHNA"
  Constant3/1 -> Sum3/2
  Sum3/1 -> Saturation1/1  "ADH"
  PA1/1 -> Saturation2/1
  Saturation1/1 -> ADH/1  "ADH"
  CNA/1 -> Sum/1

== system myGuyton_corrected_new/ADH/ADH Concentration ==
  ADH : Inport
  IC_ADHC : Constant  Value=ADHC_IC
  Integrator : Integrator  InitialConditionSource=external
  Sum : Sum  Inputs=|+-
  ain : Gain  Gain=1/ADHTC
  ADHC : Outport
  wires:
  Sum/1 -> ain/1
  ain/1 -> Integrator/1
  Integrator/1 -> Sum/2, ADHC/1  "ADHC"
  IC_ADHC/1 -> Integrator/2
  ADH/1 -> Sum/1

== system myGuyton_corrected_new/ADH/ADHMK = ADH EFFECT ON SODIUM AND  WATER REABSORPTION ==
  note: ADHKUL-1
  note: ADHZ
  note: NUM = ADHKUL-1
  note: DEN
  ADHC : Inport
  ADHKLL : Saturate  UpperLimit=inf  LowerLimit=ADHKLL
  Constant{,1..3} (4 alike) : Constant
  Divide : Product  Inputs=*/  OutScaling=2^-10
  Divide1 : Product  Inputs=/*  OutScaling=2^-10
  IC_ADHC1 : Constant  Value=ADHKLL
  IC_ADHC2 : Constant  Value=ADHKUL
  Product : Product  RndMeth=Zero
  Sum : Sum  Inputs=-+|
  Sum{1..4} (4 alike) : Sum  Inputs=|+-
  Sum5 : Sum  Inputs=|++
  ADHMK : Outport
  wires:
  Constant1/1 -> Sum1/2
  IC_ADHC2/1 -> Sum/1, Sum3/1, Sum4/1  "ADHKUL"
  Constant/1 -> Sum4/2
  Sum4/1 -> Divide/1
  Sum/1 -> Divide1/1
  IC_ADHC1/1 -> Sum/2, Sum2/1
  Divide1/1 -> Product/1  "(ADHKLL-1)/ADHZ"
  Product/1 -> Sum5/1
  Constant2/1 -> Sum5/2
  Sum5/1 -> Divide/2
  Divide/1 -> Sum3/2
  Sum3/1 -> ADHKLL/1  "ADHMK"
  Sum1/1 -> Product/2  "ADHC-1"
  ADHKLL/1 -> ADHMK/1
  ADHC/1 -> Sum1/1
  Constant3/1 -> Sum2/2
  Sum2/1 -> Divide1/2  "ADHKLL-1"

== system myGuyton_corrected_new/ADH/ADHMV = ADH EFFECT ON NONRENAL  VASCULAR RESISTANCE ==
  note: ADHVUL-1
  note: ADHZ2
  note: NUM = ADHVUL-1
  note: DEN
  ADHC : Inport
  ADHVLL : Saturate  UpperLimit=inf  LowerLimit=ADHVLL
  Constant{1..4} (4 alike) : Constant
  Divide2 : Product  Inputs=*/  OutScaling=2^-10
  Divide3 : Product  Inputs=/*  OutScaling=2^-10
  IC_ADHC1 : Constant  Value=ADHVUL
  IC_ADHC5 : Constant  Value=ADHVLL
  Product1 : Product  RndMeth=Zero
  Sum{1..2,7..8} (4 alike) : Sum  Inputs=|+-
  Sum6 : Sum  Inputs=-+|
  Sum9 : Sum  Inputs=|++
  ADHMV : Outport
  wires:
  IC_ADHC1/1 -> Sum6/1, Sum7/1, Sum8/1  "ADHVUL"
  Constant3/1 -> Sum8/2
  Sum8/1 -> Divide2/1
  Sum6/1 -> Divide3/1
  IC_ADHC5/1 -> Sum6/2, Sum2/1
  Divide3/1 -> Product1/1  "(ADHVUL-1)/ADHZ2"
  Constant4/1 -> Sum9/2
  Sum9/1 -> Divide2/2
  Divide2/1 -> Sum7/2
  Sum7/1 -> ADHVLL/1  "ADHMV"
  Sum1/1 -> Product1/2  "ADHC-1"
  Constant1/1 -> Sum1/2
  ADHC/1 -> Sum1/1
  ADHVLL/1 -> ADHMV/1
  Constant2/1 -> Sum2/2
  Sum2/1 -> Divide3/2  "ADHVLL-1"
  Product1/1 -> Sum9/1

== system myGuyton_corrected_new/ANP/ANP ACCUMULATION  AND DESTRUCTION ==
  note: ANPC
  ANP1 : Inport
  Constant1 : Constant  Value=ANPC_IC
  Gain2 : Gain  Gain=1/ANPTC
  Integrator : Integrator  InitialConditionSource=external
  Sum4 : Sum  Inputs=|+-
  ANPC : Outport
  wires:
  Sum4/1 -> Gain2/1
  Gain2/1 -> Integrator/1
  Integrator/1 -> Sum4/2, ANPC/1
  ANP1/1 -> Sum4/1
  Constant1/1 -> Integrator/2

== system myGuyton_corrected_new/Aldosterone/AM1 ==
  AMC : Inport
  Constant11 : Constant
  Constant5 : Constant  Value=AM1UL
  Constant6 : Constant
  Constant7 : Constant  Value=AM1LL
  Constant9 : Constant
  Divide : Product  Inputs=*/  OutScaling=2^-10
  Divide2 : Product  Inputs=*/  OutScaling=2^-10
  Gain3 : Gain  Gain=AMCSNS
  Product1 : Product  RndMeth=Zero
  Sum10 : Sum  Inputs=-+|
  Sum11 : Sum  Inputs=|++
  Sum6 : Sum  Inputs=|+-
  Sum7 : Sum  Inputs=|+-
  Sum8 : Sum  Inputs=|+-
  Sum9 : Sum  Orientation=left  Inputs=-+
  AM1 : Outport
  wires:
  Constant5/1 -> Sum6/1, Sum8/1, Sum9/1  "AM1UL"
  Constant6/1 -> Sum6/2, Sum10/1
  Sum6/1 -> Divide/1  "AM1UL-1"
  Constant7/1 -> Sum9/2, Sum10/2
  Sum10/1 -> Divide2/1  "AM1LL-1"
  Sum9/1 -> Divide2/2  "AM1LL-AMIUL"
  Constant9/1 -> Sum7/2
  Sum7/1 -> Product1/2  "AMC-1"
  Divide2/1 -> Product1/1
  Product1/1 -> Gain3/1
  Gain3/1 -> Sum11/1
  Constant11/1 -> Sum11/2
  Sum11/1 -> Divide/2
  Divide/1 -> Sum8/2
  Sum8/1 -> AM1/1
  AMC/1 -> Sum7/1

== system myGuyton_corrected_new/Aldosterone/AMR1 ==
  AMRBSC : Inport
  Constant2 : Constant
  Constant3 : Constant  Value=ALDINF
  Constant4 : Constant  Value=ALDKNS
  Gain2 : Gain  Gain=AMKMUL
  Saturation : Saturate  UpperLimit=inf  LowerLimit=0
  Sum3 : Sum  Inputs=|+-
  Sum4 : Sum  Inputs=|++
  Sum5 : Sum  Inputs=|++
  Switch : Switch  Criteria=u2 > Threshold
  AMR1 : Outport
  wires:
  Constant2/1 -> Sum3/2, Sum4/2
  Sum3/1 -> Gain2/1
  Gain2/1 -> Sum4/1
  Sum4/1 -> Saturation/1  "AMR"
  Saturation/1 -> Sum5/1
  Constant3/1 -> Sum5/2
  Sum5/1 -> Switch/3  "AMR1"
  Constant4/1 -> Switch/2, Switch/1
  Switch/1 -> AMR1/1  "AMR1"
  AMRBSC/1 -> Sum3/1

== system myGuyton_corrected_new/Aldosterone/AMRBSC ==
  CKE : Inport
  ANM : Inport  Port=2
  Constant : Constant  Value=3.3
  Constant1 : Constant
  Gain : Gain  Gain=ANMALD
  Gain1 : Gain  Gain=0.909
  Product : Product  RndMeth=Zero
  Sum : Sum  Inputs=|+-
  Sum1 : Sum  Inputs=|+-
  Sum2 : Sum  Inputs=|++
  AMRBSC : Outport
  wires:
  Constant/1 -> Sum/2
  Constant1/1 -> Sum1/2, Sum2/2
  Sum1/1 -> Gain/1
  Gain/1 -> Sum2/1
  Sum/1 -> Product/1
  Sum2/1 -> Product/2
  Product/1 -> Gain1/1
  ANM/1 -> Sum1/1
  CKE/1 -> Sum/1
  Gain1/1 -> AMRBSC/1  "AMRBSC"

== system myGuyton_corrected_new/Aldosterone/Aldost. Concentration Dynamics ==
  AMR1 : Inport
  Constant : Constant  Value=AMC_IC
  Gain3 : Gain  Gain=1/AMT
  Integrator : Integrator  InitialConditionSource=external
  Sum6 : Sum  Inputs=|+-
  AMC : Outport
  wires:
  Sum6/1 -> Gain3/1
  Gain3/1 -> Integrator/1
  Integrator/1 -> Sum6/2, AMC/1  "AMC"
  AMR1/1 -> Sum6/1
  Constant/1 -> Integrator/2

== system myGuyton_corrected_new/Angiotensin/ANG Secretion Dynamics ==
  ANX : Inport
  Gain : Gain  Gain=1/ANV
  IC_ANX1 : Constant  Value=ANX1_IC
  Integrator : Integrator  InitialConditionSource=external
  Sum7 : Sum  Inputs=|+-
  ANX1 : Outport
  wires:
  Sum7/1 -> Gain/1
  Gain/1 -> Integrator/1
  IC_ANX1/1 -> Integrator/2
  Integrator/1 -> Sum7/2, ANX1/1
  ANX/1 -> Sum7/1

== system myGuyton_corrected_new/Angiotensin/ANM Calculation ==
  note: ANC-1
  note: ANM
  ANC : Inport
  Constant{6,8..9,11} (4 alike) : Constant
  Constant5 : Constant  Value=ANMUL
  Constant7 : Constant  Value=ANMLL
  Divide : Product  Inputs=*/  OutScaling=2^-10
  Divide2 : Product  Inputs=*/  OutScaling=2^-10
  Gain3 : Gain  Gain=ANCSNS
  Product1 : Product  RndMeth=Zero
  Sum10 : Sum  Inputs=-+|
  Sum11 : Sum  Inputs=|++
  Sum6 : Sum  Inputs=|+-
  Sum7 : Sum  Inputs=|+-
  Sum8 : Sum  Inputs=|+-
  Sum9 : Sum  Orientation=left  Inputs=-+
  ANM : Outport
  wires:
  Constant5/1 -> Sum6/1, Sum8/1, Sum9/1  "ANMUL"
  Constant6/1 -> Sum6/2
  Sum6/1 -> Divide/1  "ANMUL-1"
  Constant7/1 -> Sum9/2, Sum10/2
  Sum10/1 -> Divide2/1  "ANMLL-1"
  Sum9/1 -> Divide2/2  "ANMLL-ANMUL"
  Constant8/1 -> Sum10/1
  Constant9/1 -> Sum7/2
  Sum7/1 -> Product1/2
  Divide2/1 -> Product1/1
  Product1/1 -> Gain3/1
  Gain3/1 -> Sum11/1
  Constant11/1 -> Sum11/2
  Sum11/1 -> Divide/2
  Divide/1 -> Sum8/2
  Sum8/1 -> ANM/1
  ANC/1 -> Sum7/1

== system myGuyton_corrected_new/Angiotensin/Angiotensin Secretion  Due to MD Flow ==
  MDFLW3 : Inport
  Constant1 : Constant
  Constant2 : Constant
  Constant3 : Constant  Orientation=up  Value=10
  Constant4 : Constant  Value=9
  Constant5 : Constant
  Divide : Product  Inputs=*/  OutScaling=2^-10
  Divide1 : Product  Inputs=*/  OutScaling=2^-10
  Gain1 : Gain  Gain=72
  Gain2 : Gain  Gain=8
  Sum1 : Sum  Inputs=|+-
  Sum2 : Sum  Inputs=|++
  Sum3 : Sum  Inputs=-+|
  Sum4 : Sum  Inputs=|++
  Sum5 : Sum  Inputs=|-+
  if MDLW3>1 : Switch  Criteria=u2 > Threshold  Threshold=1
  ANGSCR : Outport
  wires:
  Constant1/1 -> Divide/1
  Constant2/1 -> Sum1/2, Sum2/2
  Sum1/1 -> Gain1/1
  Gain1/1 -> Sum2/1
  Sum2/1 -> Divide/2
  MDFLW3/1 -> Sum3/1, Sum1/1, if MDLW3>1/2
  Divide/1 -> if MDLW3>1/1
  Constant4/1 -> Divide1/1
  Constant5/1 -> Sum3/2, Sum4/2
  Sum3/1 -> Gain2/1
  Gain2/1 -> Sum4/1
  Sum4/1 -> Divide1/2
  Divide1/1 -> Sum5/1
  Constant3/1 -> Sum5/2
  Sum5/1 -> if MDLW3>1/3
  if MDLW3>1/1 -> ANGSCR/1  "ANGSCR"

== system myGuyton_corrected_new/Angiotensin/MDFLW3 ==
  MDFLW : Inport
  Constant : Constant  Value=MDFLW3_IC
  Gain : Gain  Gain=1/300
  Integrator : Integrator  InitialConditionSource=external
  Sum : Sum  Inputs=|+-
  MDFLW3 : Outport
  wires:
  Integrator/1 -> Sum/2, MDFLW3/1  "MDFLW3"
  Constant/1 -> Integrator/2
  Gain/1 -> Integrator/1
  Sum/1 -> Gain/1
  MDFLW/1 -> Sum/1

== system myGuyton_corrected_new/Angiotensin/Plasma ANG Concentration ==
  note: ANC
  ANPR1 : Inport
  Gain : Gain  Gain=1/ANT
  IC_ANC : Constant  Value=ANC_IC
  Integrator : Integrator  InitialConditionSource=external
  Sum7 : Sum  Inputs=|+-
  ANC : Outport
  wires:
  Sum7/1 -> Gain/1
  Gain/1 -> Integrator/1
  IC_ANC/1 -> Integrator/2
  Integrator/1 -> Sum7/2, ANC/1
  ANPR1/1 -> Sum7/1

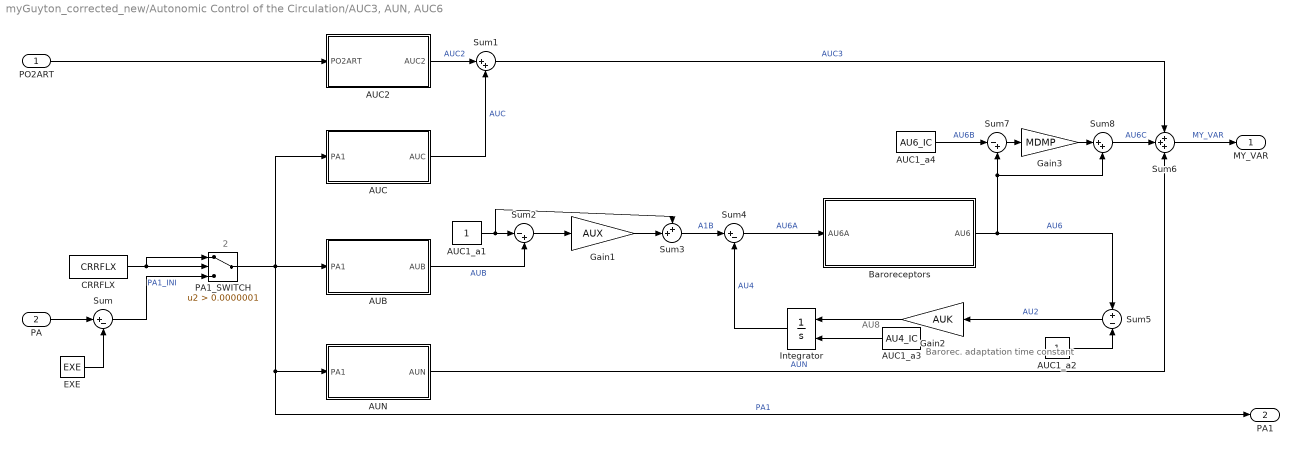
== system myGuyton_corrected_new/Autonomic Control of the Circulation/AUC3, AUN, AUC6 ==
  note: AU8
  note: Barorec. adaptation
      | time constant
  note: 2
  PO2ART : Inport
  PA : Inport  Port=2
  AUB : Subsystem
      mask Display: disp('AUB CALULATION')
  AUC : Subsystem
      mask Display: disp('AUC CALULATION')
  AUC1_a1 : Constant
  AUC1_a2 : Constant
  AUC1_a3 : Constant  Orientation=left  Value=AU4_IC
  AUC1_a4 : Constant  Value=AU6_IC
  AUC2 : Subsystem
      mask Display: disp('AUC2 CALULATION')
  AUN : Subsystem
      mask Display: disp('AUN CALULATION')
  Baroreceptors : Subsystem
      mask Display: dpoly([0 1],[BAROTC 1])
  CRRFLX : Constant  Value=CRRFLX
  EXE : Constant  Value=EXE
  Gain1 : Gain  Gain=AUX
  Gain2 : Gain  Orientation=left  Gain=AUK
  Gain3 : Gain  Gain=MDMP
  Integrator : Integrator  Orientation=left  InitialConditionSource=external
  PA1_SWITCH : Switch  Criteria=u2 > Threshold  Threshold=0.0000001
  Sum : Sum  Inputs=|+-
  Sum1 : Sum  Inputs=|++
  Sum2 : Sum  Inputs=|-+
  Sum3 : Sum  Inputs=++|
  Sum4 : Sum  Inputs=|+-
  Sum5 : Sum  Orientation=left  Inputs=+-
  Sum6 : Sum  Inputs=+++
  Sum7 : Sum  Inputs=|-+
  Sum8 : Sum  Inputs=|++
  MY_VAR : Outport
  PA1 : Outport  Port=2
  wires:
  Sum1/1 -> Sum6/1  "AUC3"
  AUN/1(AUN) -> Sum6/3  "AUN"
  Gain2/1 -> Integrator/1
  Sum5/1 -> Gain2/1  "AU2"
  AUC1_a2/1 -> Sum5/2
  Integrator/1 -> Sum4/2  "AU4"
  Baroreceptors/1(AU6) -> Sum7/2, Sum8/2, Sum5/1  "AU6"
  Sum4/1 -> Baroreceptors/1(AU6A)  "AU6A"
  AUB/1(AUB) -> Sum2/2  "AUB"
  Sum3/1 -> Sum4/1  "A1B"
  Gain1/1 -> Sum3/2
  Sum2/1 -> Gain1/1
  AUC1_a1/1 -> Sum2/1, Sum3/1
  AUC2/1(AUC2) -> Sum1/1  "AUC2"
  PA1_SWITCH/1 -> AUC/1(PA1), AUB/1(PA1), AUN/1(PA1), PA1/1  "PA1"
  AUC/1(AUC) -> Sum1/2  "AUC"
  CRRFLX/1 -> PA1_SWITCH/2, PA1_SWITCH/1
  Sum/1 -> PA1_SWITCH/3  "PA1_INI"
  EXE/1 -> Sum/2
  PA/1 -> Sum/1
  PO2ART/1 -> AUC2/1(PO2ART)
  Sum6/1 -> MY_VAR/1  "MY_VAR"
  AUC1_a3/1 -> Integrator/2
  AUC1_a4/1 -> Sum7/1  "AU6B"
  Sum7/1 -> Gain3/1
  Gain3/1 -> Sum8/1
  Sum8/1 -> Sum6/2  "AU6C"

== system myGuyton_corrected_new/Autonomic Control of the Circulation/Autonom. drive due to low pres. receptors  ==
  PRA : Inport
  PLA : Inport  Port=2
  PPA : Inport  Port=3
  Constant : Constant  Value=15
  Constant1 : Constant
  Divide : Product  Inputs=*/  OutScaling=2^-10
  Gain : Gain  Gain=AULPM
  Sum : Sum  Inputs=|+-
  Sum1 : Sum  Inputs=|++
  Sum6 : Sum  Inputs=+++
  AULP : Outport
  wires:
  Constant/1 -> Divide/1
  Sum6/1 -> Divide/2
  Constant1/1 -> Sum/2, Sum1/2
  Divide/1 -> Sum/1
  Sum/1 -> Gain/1
  Gain/1 -> Sum1/1
  PRA/1 -> Sum6/1
  PPA/1 -> Sum6/3
  Sum1/1 -> AULP/1
  PLA/1 -> Sum6/2

== system myGuyton_corrected_new/Autonomic Control of the Circulation/Subsystem1 ==
  AUTTL : Inport
  Constant3 : Constant  Value=AUMAX
  Constant6 : Constant
  Constant7 : Constant  Orientation=up
  Divide : Product  Inputs=*/  OutScaling=2^-10
  Gain1 : Gain  Gain=AUSLP
  Saturation1 : Saturate  UpperLimit=inf  LowerLimit=AUMIN  LinearizeAsGain=off
  Subsystem3 : Subsystem
      mask Display: dpoly([0 1],[AUDMP 1])
  Sum2 : Sum  Inputs=|+-
  Sum3 : Sum  Inputs=|+-
  Sum4 : Sum  Inputs=|+-
  exp(AUSLP*(AU1-1)) : Math  SaturateOnIntegerOverflow=on
  AU : Outport
  wires:
  Subsystem3/1(AU1) -> Sum4/1  "AU1"
  Constant3/1 -> Sum2/1, Sum3/1  "AUMAX"
  Constant6/1 -> Sum3/2
  Sum3/1 -> Divide/1  "AUMAX-1"
  Constant7/1 -> Sum4/2
  Sum4/1 -> Gain1/1  "AU1-1"
  Gain1/1 -> exp(AUSLP*(AU1-1))/1
  exp(AUSLP*(AU1-1))/1 -> Divide/2
  Divide/1 -> Sum2/2
  Sum2/1 -> Saturation1/1
  Saturation1/1 -> AU/1
  AUTTL/1 -> Subsystem3/1(AUTTL)

== system myGuyton_corrected_new/Autoregulation/Muscle Local BF Control ==
  PMO : Inport
  AMM4 : Saturate  UpperLimit=inf  LowerLimit=AMM4  LinearizeAsGain=off
  ARM12 : Product  RndMeth=Nearest
  ARM2 : Gain  Gain=POM
  ARM8 : Gain  Gain=POM2
  Constant : Constant  Value=38
  Constant1 : Constant
  Constant2 : Constant
  Long-Term Muscle Auotoreg. : Subsystem
      mask Display: dpoly([0 1],[A4K2 1])
  Rapid Muscle Autoregulation : Subsystem
      mask Display: dpoly([0 1],[A4K 1])
  Sum : Sum  Inputs=|+-
  Sum1 : Sum  Inputs=|++
  Sum3 : Sum  Inputs=|++
  AMM : Outport
  wires:
  Constant/1 -> Sum/2
  Sum/1 -> ARM2/1, ARM8/1  "PDO"
  ARM2/1 -> Sum1/1
  Sum1/1 -> Rapid Muscle Autoregulation/1(POE)  "POE"
  Sum3/1 -> Long-Term Muscle Auotoreg./1(In1)
  ARM8/1 -> Sum3/1
  Constant1/1 -> Sum1/2
  Constant2/1 -> Sum3/2
  Rapid Muscle Autoregulation/1(AMM1) -> AMM4/1  "AMM1"
  Long-Term Muscle Auotoreg./1(AMM2) -> ARM12/2  "AMM2"
  AMM4/1 -> ARM12/1
  ARM12/1 -> AMM/1
  PMO/1 -> Sum/1

== system myGuyton_corrected_new/Autoregulation/Non-Muscle Local BF Control ==
  POT : Inport
  ARN13A : Saturate  UpperLimit=inf  LowerLimit=0.5  LinearizeAsGain=off
  ARN14 : Gain  Gain=POZ
  ARN{3,9,15,19,21} (5 alike) : Constant
  ARN17A : Saturate  UpperLimit=inf  LowerLimit=0.3  LinearizeAsGain=off
  ARN18 : Product  Inputs=3  RndMeth=Zero
  ARN2 : Gain  Gain=POK
  ARN20 : Gain  Gain=AUTOSN
  ARN7A : Saturate  UpperLimit=inf  LowerLimit=0.5  LinearizeAsGain=off
  ARN8 : Gain  Gain=PON
  Constant : Constant  Value=POR
  Intermediate Autoreg. : Subsystem
      mask Display: dpoly([0 1],[ A2K 1],'s')
  Long-Term Autoreg. : Subsystem
      mask Display: dpoly([0 1],[A3K 1],'s')
  Rapid Autoreg. : Subsystem
      mask Display: dpoly([0 1],[A1K 1],'s')
  Sum : Sum  Inputs=|+-
  Sum{1..3,8} (4 alike) : Sum  Inputs=|++
  Sum7 : Sum  Inputs=|+-
  ARM : Outport
  wires:
  Constant/1 -> Sum/2
  Sum/1 -> ARN8/1, ARN14/1, ARN2/1  "POD"
  ARN14/1 -> Sum1/1
  ARN15/1 -> Sum1/2
  ARN8/1 -> Sum2/1
  ARN9/1 -> Sum2/2
  ARN2/1 -> Sum3/1
  ARN3/1 -> Sum3/2
  ARN17A/1 -> ARN18/1  "AR3"
  ARN13A/1 -> ARN18/2  "AR2"
  ARN7A/1 -> ARN18/3  "AR1"
  ARN19/1 -> Sum7/2
  ARN18/1 -> Sum7/1
  Sum7/1 -> ARN20/1
  ARN21/1 -> Sum8/2
  ARN20/1 -> Sum8/1
  Sum1/1 -> Long-Term Autoreg./1(POC)  "POC"
  Sum2/1 -> Intermediate Autoreg./1(POA)  "POA"
  Sum3/1 -> Rapid Autoreg./1(POB)  "POB"
  Long-Term Autoreg./1(AR3) -> ARN17A/1  "AR3"
  Intermediate Autoreg./1(AR2) -> ARN13A/1  "AR2"
  Rapid Autoreg./1(AR1) -> ARN7A/1  "AR1"
  POT/1 -> Sum/1
  Sum8/1 -> ARM/1

== system myGuyton_corrected_new/CIRCULATION/Damping ==
  QLO : Inport  Orientation=down
  QPO_a : Inport  Orientation=left  Port=2
  CD5 : Product  Orientation=left  Inputs=*/  OutScaling=2^-10
  Constant12 : Constant  Orientation=left  Value=U
  Sum1 : Sum  Orientation=left  Inputs=++|
  Sum18 : Sum  Orientation=left  Inputs=-+|
  QPO : Outport  Orientation=left
  wires:
  Constant12/1 -> CD5/2
  Sum18/1 -> CD5/1
  QLO/1 -> Sum18/1, Sum1/1
  QPO_a/1 -> Sum18/2
  CD5/1 -> Sum1/2
  Sum1/1 -> QPO/1

== system myGuyton_corrected_new/CIRCULATION/Damping1 ==
  QRO : Inport  Orientation=left
  QVO_a : Inport  Orientation=left  Port=2
  CD5 : Product  Orientation=left  Inputs=*/  OutScaling=2^-10
  Constant12 : Constant  Orientation=left  Value=X
  Sum1 : Sum  Orientation=left  Inputs=++|
  Sum18 : Sum  Orientation=left  Inputs=-+|
  QVO : Outport  Orientation=left
  wires:
  Constant12/1 -> CD5/2
  Sum18/1 -> CD5/1
  QRO/1 -> Sum18/1, Sum1/1
  CD5/1 -> Sum1/2
  Sum1/1 -> QVO/1
  QVO_a/1 -> Sum18/2

== system myGuyton_corrected_new/CIRCULATION/FUN1 ==
  PA2 : Inport  Orientation=left
  FUN1 : simulink/Lookup Tables/Lookup Table (n-D)  Orientation=left  numDimsPopupSelect=1  bp1="[0,  60 , 125,  160, 200, 240 ]"  bp2=[10,22,31]  bp3=[1:3]  bp4=[1:3]  bpcell={ [1:3], [1:3] }  explicitNumDims=2  searchMode=Binary Search  cacheBpFlag=off  vectorInputFlag=off  tableData=[1.04, 1.025, 0.97, 0.88, 0.59, 0]  interpMethod=Cubic Spline  extrapMethod=None - Clip  rangeErrorMode=None
  LVM : Outport  Orientation=left
  wires:
  PA2/1 -> FUN1/1
  FUN1/1 -> LVM/1  "LVM"

== system myGuyton_corrected_new/CIRCULATION/FUN3 ==
  PP2 : Inport
  FUN3 : simulink/Lookup Tables/Lookup Table (n-D)  numDimsPopupSelect=1  bp1="[0,  32, 38.4, 48.0, 60.8, 72.0]"  bp2=[10,22,31]  bp3=[1:3]  bp4=[1:3]  bpcell={ [1:3], [1:3] }  explicitNumDims=2  searchMode=Binary Search  cacheBpFlag=off  vectorInputFlag=off  tableData="[1.06,  0.97,   0.93,  0.8,  0.46,  0.0]"  interpMethod=Cubic Spline  extrapMethod=None - Clip  rangeErrorMode=None
  RVM : Outport
  wires:
  PP2/1 -> FUN3/1
  FUN3/1 -> RVM/1  "RVM"

== system myGuyton_corrected_new/CIRCULATION/FUN4 ==
  PLA1 : Inport  Orientation=up
  fun4 : simulink/Lookup Tables/Lookup Table (n-D)  Orientation=up  numDimsPopupSelect=1  bp1=[-2, 1, 5, 8, 12]  bp2=[10,22,31]  bp3=[1:3]  bp4=[1:3]  bpcell={ [1:3], [1:3] }  explicitNumDims=2  searchMode=Binary Search  cacheBpFlag=off  vectorInputFlag=off  tableData=[0.01, 3.6, 9.4, 11.6, 13.5]  interpMethod=Cubic Spline  extrapMethod=Cubic Spline  rangeErrorMode=None
  QLN : Outport  Orientation=up
  wires:
  fun4/1 -> QLN/1  "QLN"
  PLA1/1 -> fun4/1

== system myGuyton_corrected_new/CIRCULATION/MYOGRS Calculation ==
  TENS1 : Inport
  CD10 : Product  Inputs=/*  OutScaling=2^-10
  CD9 : Product  Inputs=*/  OutScaling=2^-10
  Constant1 : Constant  Value=RAD_IC
  Constant24 : Constant  Value=TENSGN
  Constant{26..29} (4 alike) : Constant
  Constant30 : Constant  Value=4
  Gain24 : Gain  Gain=1/TENSTC
  Integrator5 : Integrator  InitialConditionSource=external
  Math Function4 : Math  Operator=pow  SaturateOnIntegerOverflow=on
  Product11 : Product  RndMeth=Zero
  Sum37 : Sum  Inputs=|+-
  Sum38 : Sum  Inputs=++|
  Sum39 : Sum  Inputs=|++
  Sum40 : Sum  Inputs=+-
  Switch1 : Switch  Criteria=u2 > Threshold
  MYOGRS : Outport
  wires:
  TENS1/1 -> Product11/1, Sum37/1
  Constant26/1 -> Sum37/2, Sum38/1
  Sum37/1 -> CD9/1
  Constant24/1 -> Sum38/2, Switch1/2  "TENSGN"
  Sum38/1 -> CD9/2
  CD9/1 -> Sum39/1
  Constant27/1 -> Sum39/2
  Sum39/1 -> Sum40/1  "TENS2"
  Product11/1 -> Sum40/2  "TENS"
  Sum40/1 -> Gain24/1  "TENS2-TENS"
  Constant29/1 -> CD10/2
  CD10/1 -> Math Function4/1
  Constant30/1 -> Math Function4/2
  Math Function4/1 -> Switch1/1  "MYOGRS"
  Constant28/1 -> Switch1/3
  Switch1/1 -> MYOGRS/1
  Integrator5/1 -> Product11/2, CD10/1  "RAD"
  Constant1/1 -> Integrator5/2
  Gain24/1 -> Integrator5/1

== system myGuyton_corrected_new/CIRCULATION/PAMK Calculation ==
  PA/100 : Inport
  Constant33 : Constant
  Gain24 : Gain  Gain=KORGN
  PAMK DYNAMICS : Subsystem
      mask Display: dpoly([0 1],[KORTC 1])
  Sum41 : Sum  Inputs=|+-
  Sum42 : Sum  Inputs=|++
  PAMK : Outport
  wires:
  Constant33/1 -> Sum41/2, Sum42/2
  Sum41/1 -> Gain24/1
  Gain24/1 -> Sum42/1
  Sum42/1 -> PAMK DYNAMICS/1(In1)
  PA/100/1 -> Sum41/1
  PAMK DYNAMICS/1(PAMK) -> PAMK/1

== system myGuyton_corrected_new/CIRCULATION/QRN Calculation (FUN2) ==
  PRA : Inport  Orientation=down
  AU : Inport  Orientation=left  Port=2
  Constant8 : Constant  Orientation=left  Value=8
  Constant9 : Constant  Orientation=left
  FUN2 : Subsystem  Orientation=left
      mask Display: plot([-8, -6, -2, 4, 12],[0, 0.75, 2.6, 9.8, 13.5])
  Gain9 : Gain  Orientation=left  Gain=HTAUML
  Product5 : Product  Orientation=left  RndMeth=Zero
  Sum11 : Sum  Orientation=left
  Sum12 : Sum  Orientation=left  Inputs=|+-
  Sum13 : Sum  Orientation=left  Inputs=|++
  Sum14 : Sum  Orientation=left  Inputs=|+-
  QRN : Outport  Orientation=left
  wires:
  Constant8/1 -> Sum11/2, Sum14/2
  Sum11/1 -> Product5/1
  AU/1 -> Sum12/1
  Constant9/1 -> Sum12/2, Sum13/2
  Sum12/1 -> Gain9/1
  Gain9/1 -> Sum13/1
  Sum13/1 -> Product5/2
  Product5/1 -> Sum14/1
  Sum14/1 -> FUN2/1(PRA1)  "PRA1"
  PRA/1 -> Sum11/1
  FUN2/1(QRN) -> QRN/1  "QRN"

== system myGuyton_corrected_new/CIRCULATION/RMULT1 Calculation ==
  BFN : Inport  Orientation=down
  BFM : Inport  Orientation=up  Port=2
  CD11 : Product  Inputs=*/  OutScaling=2^-10
  Constant1 : Constant
  Constant34 : Constant  Value=AUTO
  Constant36 : Constant  Value=3.8
  Constant37 : Constant  Orientation=up
  Gain24 : Gain  Gain=AUTOGN
  Subsystem : Subsystem
      mask Display: dpoly([0 1],[1/AUTOK 1])
  Sum41 : Sum
  Sum42 : Sum  Inputs=|+-
  Sum43 : Sum  Inputs=|++
  Switch4 : Switch  Criteria=u2 > Threshold
  RMULT1 : Outport
  wires:
  Sum41/1 -> CD11/1
  Constant36/1 -> CD11/2
  CD11/1 -> Sum42/1
  Constant37/1 -> Sum42/2, Sum43/2
  Sum42/1 -> Gain24/1
  Gain24/1 -> Sum43/1
  Sum43/1 -> Subsystem/1(In1)  "RMULT"
  BFN/1 -> Sum41/1
  BFM/1 -> Sum41/2
  Constant34/1 -> Switch4/2
  Switch4/1 -> RMULT1/1
  Constant1/1 -> Switch4/3
  Subsystem/1(Out1) -> Switch4/1

== system myGuyton_corrected_new/CIRCULATION/RPA Calculation ==
  PPA : Inport  Orientation=left
  CD62 : Product  Orientation=left  Inputs=*/  OutScaling=2^-10
  Constant14 : Constant  Orientation=left
  Constant15 : Constant  Value=0.5
  Gain14 : Gain  Orientation=left  Gain=0.026
  Math Function1 : Math  Orientation=left  Operator=pow  SaturateOnIntegerOverflow=on
  Saturation3 : Saturate  Orientation=left  UpperLimit=inf  LowerLimit=0.00001
  RPA : Outport  Orientation=left
  wires:
  Math Function1/1 -> CD62/2  "CPA"
  Constant15/1 -> Math Function1/2
  Saturation3/1 -> Math Function1/1  "PP1"
  Gain14/1 -> Saturation3/1
  Constant14/1 -> CD62/1
  PPA/1 -> Gain14/1
  CD62/1 -> RPA/1  "RPA"
